simulink model "digitalControlTustinSim"  (R2020a)
settings: Solver=VariableStepAuto  StartTime=0.0  StopTime=120  RelTol=1e-6
values from neighbouring files (symbols this model uses):
  Kp = 14.029    [digitalControlSyntesis.m]
  T = 1    [backwardDiscretization.m]    (also in backwardDiscretizationMultipleT.m = Tvec(k); digitalControlSyntesis.m = 0.1; discretizacion.m = Tvec(k); tustinDiscretization.m)
  Td = 12.5    [digitalControlSyntesis.m]
  Ti = 13.5593    [digitalControlSyntesis.m]
undefined symbols (not defined in the file or in its folder): den_tust, num_tust
libraries: simulink x1
settings Model: Creator=gbecerra  LastModifiedBy=gbecerra

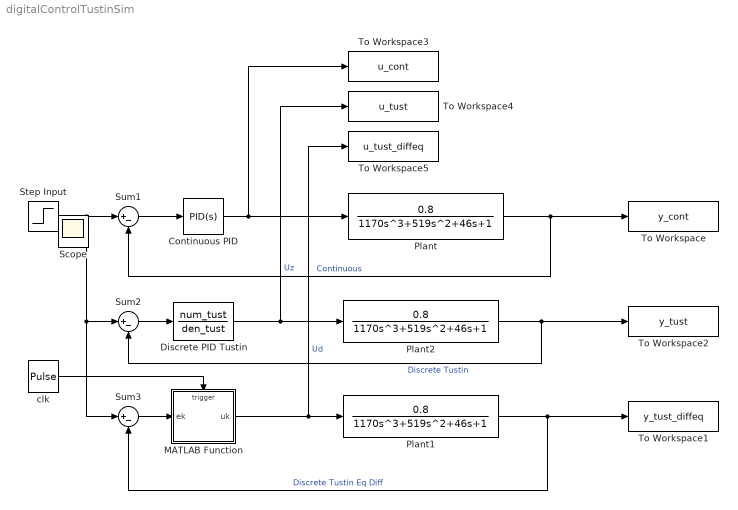
== system digitalControlTustinSim ==
  Continuous PID : simulink/Continuous/PID Controller  Controller=PID  Form=Ideal  TimeDomain=Continuous-time  UseExternalTs=off  SampleTime=-1  IntegratorMethod=Forward Euler  FilterMethod=Forward Euler  ControllerParametersSource=internal  P=Kp  I=1/Ti  D=Td  UseFilter=on  N=100  TunerSelectOption=Transfer Function Based (PID Tuner App)  InitialConditionSource=internal  InitialConditionForIntegrator=0  InitialConditionForFilter=0  DifferentiatorICPrevScaledInput=0  ExternalReset=none  TrackingMode=off  Kt=1  LimitOutput=off  UpperSaturationLimit=inf  LowerSaturationLimit=-inf  LinearizeAsGain=on  AntiWindupMode=none  Kb=1  POutMin=[]  POutMax=[]  IOutMin=[]  IOutMax=[]  DOutMin=[]  DOutMax=[]  NOutMin=[]  NOutMax=[]  SumOutMin=[]  SumOutMax=[]  SaturationOutMin=[]  SaturationOutMax=[]  PParamMin=[]  PParamMax=[]  IParamMin=[]  IParamMax=[]  DParamMin=[]  DParamMax=[]  NParamMin=[]  NParamMax=[]  KbParamMin=[]  KbParamMax=[]  KtParamMin=[]  KtParamMax=[]  KbOutMin=[]  KbOutMax=[]  KtOutMin=[]  KtOutMax=[]  IntegratorOutMin=[]  IntegratorOutMax=[]  FilterOutMin=[]  FilterOutMax=[]  SumI1OutMin=[]  SumI1OutMax=[]  SumI2OutMin=[]  SumI2OutMax=[]  SumI3OutMin=[]  SumI3OutMax=[]  SumI4OutMin=[]  SumI4OutMax=[]  SumDOutMin=[]  SumDOutMax=[]  DifferentiatorOutMin=[]  DifferentiatorOutMax=[]  FilterDiffOutCoefMin=[]  FilterDiffOutCoefMax=[]  ReciprocalOutMin=[]  ReciprocalOutMax=[]  SumDenOutMin=[]  SumDenOutMax=[]  SumNumOutMin=[]  SumNumOutMax=[]  DivideOutMin=[]  DivideOutMax=[]  UdiffTsProdOutMin=[]  UdiffTsProdOutMax=[]  NTsProdOutMin=[]  NTsProdOutMax=[]  UintegralTsProdOutMin=[]  UintegralTsProdOutMax=[]  UngainTsProdOutMin=[]  UngainTsProdOutMax=[]  IntegratorContinuousStateAttributes=''  IntegratorStateMustResolveToSignalObject=off  IntegratorRTWStateStorageClass=Auto  FilterContinuousStateAttributes=''  FilterStateMustResolveToSignalObject=off  FilterRTWStateStorageClass=Auto  ParallelPVariant=Passthrough  IdealPVariant=InternalParameters  IVariant=InternalParameters  DVariant=InternalParameters  IntegratorVariant=Continuous  SatVariant=Disabled  AWVariant=Passthrough  PCopyVariant=Disabled  TRVariant=Disabled  FdbkBlocksVariant=Forward  IdealPFdbkVariant=Disabled  SatFdbkVariant=Disabled  DerivativeFilterVariant=ContFilter  NVariant=InternalParameters  NCopyVariant=Disabled  FilterICVariant=InternalICsFilter  IntegratorICVariant=InternalICs  ExternalResetVariant=Disabled  TRSumVariant=Passthrough  SumFdbkVariant=Disabled  SumVariant=Sum_PID  TsampFilterVariant=InternalTs  TsampNgainVariant=Passthrough  TsampIntegralVariant=Passthrough
  Discrete PID Tustin : DiscreteTransferFcn  Numerator=num_tust  Denominator=den_tust  SampleTime=T
  MATLAB Function : MATLAB Function  TreatAsAtomicUnit=on
  Plant : TransferFcn  Numerator=0.8  Denominator=[1170 519 46 1]
  Plant1 : TransferFcn  Numerator=0.8  Denominator=[1170 519 46 1]
  Plant2 : TransferFcn  Numerator=0.8  Denominator=[1170 519 46 1]
  Step Input : Step  Time=0  SampleTime=0
  Sum1 : Sum  Inputs=|+-
  Sum2 : Sum  Inputs=|+-
  Sum3 : Sum  Inputs=|+-
  To Workspace : ToWorkspace  VariableName=y_cont  SaveFormat=Timeseries  SampleTime=-1
  To Workspace1 : ToWorkspace  VariableName=y_tust_diffeq  SaveFormat=Timeseries  SampleTime=-1
  To Workspace2 : ToWorkspace  VariableName=y_tust  SaveFormat=Timeseries  SampleTime=-1
  To Workspace3 : ToWorkspace  VariableName=u_cont  SaveFormat=Timeseries  SampleTime=-1
  To Workspace4 : ToWorkspace  VariableName=u_tust  SaveFormat=Timeseries  SampleTime=-1
  To Workspace5 : ToWorkspace  VariableName=u_tust_diffeq  SaveFormat=Timeseries  SampleTime=-1
  clk : DiscretePulseGenerator  PulseType=Time based  Period=T  PulseWidth=50  PhaseDelay=1e-9
  Scope : Scope
  wires:
  Step Input/1 -> Sum3/1, Sum2/1, Sum1/1
  Plant/1 -> Sum1/2, To Workspace/1  "Continuous"
  Sum1/1 -> Continuous PID/1
  Sum2/1 -> Discrete PID Tustin/1
  Discrete PID Tustin/1 -> To Workspace4/1, Plant2/1  "Uz"
  Plant2/1 -> To Workspace2/1, Sum2/2  "Discrete Tustin"
  Plant1/1 -> Sum3/2, To Workspace1/1  "Discrete Tustin Eq Diff"
  Sum3/1 -> MATLAB Function/1(ek)
  clk/1 -> MATLAB Function/Trigger
  MATLAB Function/1(uk) -> Plant1/1, To Workspace5/1  "Ud"
  Continuous PID/1 -> To Workspace3/1, Plant/1

== matlab function digitalControlTustinSim/MATLAB Function ==
  data: ek input; uk output; num_tust parameter; den_tust parameter
  events: clock input RISING_EDGE_EVENT
function uk = diffeq(ek,num_tust,den_tust)
persistent ek1      % e(k-1)
persistent ek2      % e(k-2)
persistent uk1      % u(k-1)
persistent uk2      % u(k-2)
if isempty(ek1) && isempty(ek2) && isempty(uk1) && isempty(uk2)
    ek1 = 0; ek2 = 0;   % Initializes persistent variables
    uk1 = 0; uk2 = 0;   % during the first execution
end
b2 = num_tust(1);
b1 = num_tust(2);   % Configures coefficients in the
b0 = num_tust(3);   % difference equation
a2 = den_tust(1);
a1 = den_tust(2);
a0 = den_tust(3); 
% Computes the current iteration of the difference equation
uk = -(a0/a2)*uk2 + (b2/a2)*ek + (b1/a2)*ek1 + (b0/a2)*ek2;
% Shifts the values in e and u for the next iteration
% e(k-2) <- e(k-1), e(k-1) <- e(k)
% u(k-2) <- u(k-1), u(k-1) <- u(k), 
ek2 = ek1; ek1 = ek; uk2 = uk1; uk1 = uk;
